simulink model "Pre4"  (R2015b)
settings: Solver=ode3  StartTime=0.0  StopTime=5  FixedStep=0.01  RelTol=1e-3
undefined symbols (not defined in the file): K, Kd
settings Model: Creator=FANUC  LastModifiedBy=FANUC
settings DataIOCC: LimitDataPoints=off  SaveFormat=Array  TimeSaveName=t  OutputSaveName=x

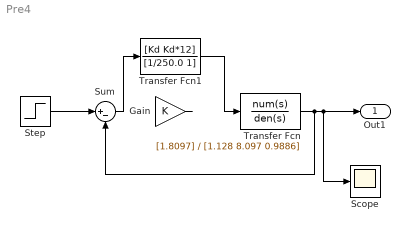
== system Pre4 ==
  Gain : Gain  Gain=K
  Scope : Scope
  Step : Step  Time=0  SampleTime=0
  Sum : Sum  Inputs=|+-
  Transfer Fcn : TransferFcn  Numerator=[1.8097]  Denominator=[1.128 8.097 0.9886]
  Transfer Fcn1 : TransferFcn  Numerator=[Kd Kd*12]  Denominator=[1/250.0 1]
  Out1 : Outport
  wires:
  Step/1 -> Sum/1
  Sum/1 -> Transfer Fcn1/1
  Gain/1 -> ?
  Transfer Fcn/1 -> Sum/2, Scope/1, Out1/1
  Transfer Fcn1/1 -> Transfer Fcn/1
